simulink model "mc_pos"  (R2021a)
settings: Solver=FixedStepAuto  StartTime=0.0  StopTime=10.0  FixedStep=0.1  RelTol=1e-3
undefined symbols (not defined in the file): CONSTANTS_ONE_G, DiscIntNeverNeededParam, MPC_LAND_SPEED, MPC_SPOOLUP_TIME, MPC_THR_HOVER, MPC_THR_MAX, MPC_THR_MIN, MPC_TILTMAX_AIR, MPC_TILTMAX_LND, MPC_TKO_RAMP_T, MPC_VELD_LP, MPC_XY_P, MPC_XY_VEL_D_ACC, MPC_XY_VEL_I_ACC, MPC_XY_VEL_MAX, MPC_XY_VEL_P_ACC, MPC_Z_P, MPC_Z_VEL_D_ACC, MPC_Z_VEL_I_ACC, MPC_Z_VEL_MAX_DN, MPC_Z_VEL_MAX_UP, MPC_Z_VEL_P_ACC, PX4_TAKEOFF_STATUS, WV_EN
libraries: simulink x16, vrlib x2, sharedtransform x2, aerolibconvert2 x1
(part 1 of 3)
settings Model: DataDictionary=px4_dict.sldd  Creator=DELL  LastModifiedBy=yu
settings OptimizationCC: DefaultParameterBehavior=Inlined  EnhancedBackFolding=on  PassReuseOutputArgsAs=Individual arguments  ZeroExternalMemoryAtStartup=off  ZeroInternalMemoryAtStartup=off  OptimizeBlockOrder=speed  DifferentSizesBufferReuse=on  OptimizationCustomize=off  EfficientTunableParamExpr=on
settings DebuggingCC: ParameterTunabilityLossMsg=error
settings SFSimCC: MATLABDynamicMemAlloc=off
settings RTWCC: SystemTargetFile=ert.tlc  TemplateMakefile=ert_default_tmf
settings CodeAppCC: ForceParamTrailComments=on  IgnoreCustomStorageClasses=off  OperatorAnnotations=on  SimulinkDataObjDesc=on  SFDataObjDesc=on  InsertBlockDesc=on
settings ERTTargetCC: TargetLangStandard=C99 (ISO)  GenerateSampleERTMain=on  SupportContinuousTime=on  InlinedParameterPlacement=NonHierarchical  ERTCustomFileTemplate=example_file_process.tlc

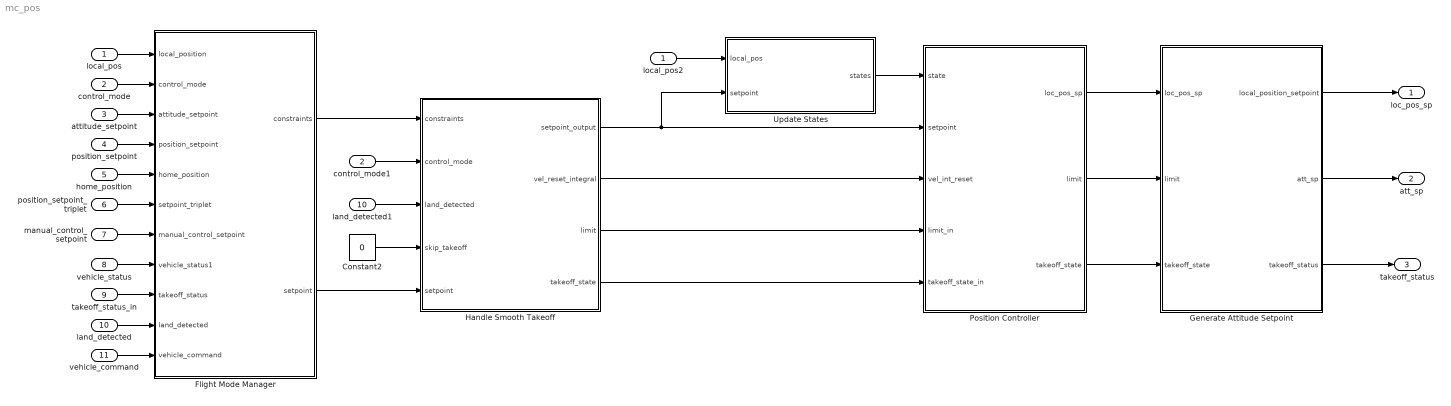
== system mc_pos ==
  local_pos : Inport  OutDataTypeStr=Bus: px4_vehicle_local_position
  control_mode : Inport  Port=2  OutDataTypeStr=Bus: px4_vehicle_control_mode
  attitude_setpoint : Inport  Port=3  OutDataTypeStr=Bus: px4_vehicle_attitude_setpoint
  position_setpoint : Inport  Port=4  OutDataTypeStr=Bus: px4_vehicle_local_position_setpoint
  home_position : Inport  Port=5  OutDataTypeStr=Bus: px4_home_position
  position_setpoint_triplet : Inport  Port=6  OutDataTypeStr=Bus: px4_position_setpoint_triplet
  manual_control_setpoint : Inport  Port=7  OutDataTypeStr=Bus: px4_manual_control_setpoint
  vehicle_status : Inport  Port=8  OutDataTypeStr=Bus: px4_vehicle_status
  takeoff_status_in : Inport  Port=9  OutDataTypeStr=Bus: px4_takeoff_status
  land_detected : Inport  Port=10  OutDataTypeStr=Bus: px4_vehicle_land_detected
  vehicle_command : Inport  Port=11  OutDataTypeStr=Bus: px4_vehicle_command
  Constant2 : Constant  Value=0  OutDataTypeStr=boolean
  Flight Mode Manager : Subsystem
  Generate Attitude Setpoint : Subsystem
  Handle Smooth Takeoff : Stateflow chart  TreatAsAtomicUnit=on
  Position Controller : Subsystem
  Update States : Subsystem
  control_mode1 : InportShadow  Port=2  OutDataTypeStr=Bus: px4_vehicle_control_mode
  land_detected1 : InportShadow  Port=10  OutDataTypeStr=Bus: px4_vehicle_land_detected
  local_pos2 : InportShadow  OutDataTypeStr=Bus: px4_vehicle_local_position
  loc_pos_sp : Outport  OutDataTypeStr=Bus: px4_vehicle_local_position_setpoint  BusOutputAsStruct=on
  att_sp : Outport  Port=2  OutDataTypeStr=Bus: px4_vehicle_attitude_setpoint  BusOutputAsStruct=on
  takeoff_status : Outport  Port=3  OutDataTypeStr=Bus: px4_takeoff_status  BusOutputAsStruct=on
  wires:
  local_pos/1 -> Flight Mode Manager/1(local_position)
  Flight Mode Manager/2(setpoint) -> Handle Smooth Takeoff/5(setpoint)
  Update States/1(states) -> Position Controller/1(state)
  Position Controller/1(loc_pos_sp) -> Generate Attitude Setpoint/1(loc_pos_sp)
  land_detected1/1 -> Handle Smooth Takeoff/3(land_detected)
  Flight Mode Manager/1(constraints) -> Handle Smooth Takeoff/1(constraints)
  Constant2/1 -> Handle Smooth Takeoff/4(skip_takeoff)
  Handle Smooth Takeoff/1(setpoint_output) -> Update States/2(setpoint), Position Controller/2(setpoint)
  Handle Smooth Takeoff/3(limit) -> Position Controller/4(limit_in)
  Handle Smooth Takeoff/2(vel_reset_integral) -> Position Controller/3(vel_int_reset)
  control_mode/1 -> Flight Mode Manager/2(control_mode)
  land_detected/1 -> Flight Mode Manager/10(land_detected)
  position_setpoint/1 -> Flight Mode Manager/4(position_setpoint)
  home_position/1 -> Flight Mode Manager/5(home_position)
  position_setpoint_triplet/1 -> Flight Mode Manager/6(setpoint_triplet)
  manual_control_setpoint/1 -> Flight Mode Manager/7(manual_control_setpoint)
  vehicle_status/1 -> Flight Mode Manager/8(vehicle_status1)
  Generate Attitude Setpoint/2(att_sp) -> att_sp/1
  attitude_setpoint/1 -> Flight Mode Manager/3(attitude_setpoint)
  takeoff_status_in/1 -> Flight Mode Manager/9(takeoff_status)
  local_pos2/1 -> Update States/1(local_pos)
  vehicle_command/1 -> Flight Mode Manager/11(vehicle_command)
  control_mode1/1 -> Handle Smooth Takeoff/2(control_mode)
  Position Controller/2(limit) -> Generate Attitude Setpoint/2(limit)
  Handle Smooth Takeoff/4(takeoff_state) -> Position Controller/5(takeoff_state_in)
  Position Controller/3(takeoff_state) -> Generate Attitude Setpoint/3(takeoff_state)
  Generate Attitude Setpoint/3(takeoff_status) -> takeoff_status/1
  Generate Attitude Setpoint/1(local_position_setpoint) -> loc_pos_sp/1

== system mc_pos/Flight Mode Manager ==
  local_position : Inport  OutDataTypeStr=Bus: px4_vehicle_local_position
  control_mode : Inport  Port=2  OutDataTypeStr=Bus: px4_vehicle_control_mode
  attitude_setpoint : Inport  Port=3  OutDataTypeStr=Bus: px4_vehicle_attitude_setpoint
  position_setpoint : Inport  Port=4  OutDataTypeStr=Bus: px4_vehicle_local_position_setpoint
  home_position : Inport  Port=5  OutDataTypeStr=Bus: px4_home_position
  setpoint_triplet : Inport  Port=6  OutDataTypeStr=Bus: px4_position_setpoint_triplet
  manual_control_setpoint : Inport  Port=7  OutDataTypeStr=Bus: px4_manual_control_setpoint
  vehicle_status1 : Inport  Port=8  OutDataTypeStr=Bus: px4_vehicle_status
  Bus Element In : Inport  Port=9  PortName=takeoff_status  Element=takeoff_state
  Bus Element In1 : Inport  Port=9  PortName=takeoff_status  Element=takeoff_state
  land_detected : Inport  Port=10  OutDataTypeStr=Bus: px4_vehicle_land_detected
  vehicle_command : Inport  Port=11  OutDataTypeStr=Bus: px4_vehicle_command
  Flight Task : Stateflow chart  TreatAsAtomicUnit=on
  Output : Subsystem
  Weather Vane : Subsystem
  control_mode1 : InportShadow  Port=2  OutDataTypeStr=Bus: px4_vehicle_control_mode
  home_position1 : InportShadow  Port=5  OutDataTypeStr=Bus: px4_home_position
  local_position1 : InportShadow  OutDataTypeStr=Bus: px4_vehicle_local_position
  local_position2 : InportShadow  OutDataTypeStr=Bus: px4_vehicle_local_position
  vehicle_status : InportShadow  Port=8  OutDataTypeStr=Bus: px4_vehicle_status
  constraints : Outport
  setpoint : Outport  Port=2
  wires:
  home_position/1 -> Flight Task/5(home_position)
  setpoint_triplet/1 -> Flight Task/6(triplet_setpoint)
  manual_control_setpoint/1 -> Flight Task/7(manual_control_setpoint)
  vehicle_status1/1 -> Flight Task/8(vehicle_status)
  attitude_setpoint/1 -> Weather Vane/3(attitude_setpoint)
  Weather Vane/1(weather_vane) -> Flight Task/1(weather_vane)
  position_setpoint/1 -> Flight Task/2(position_setpoint_input)
  Flight Task/4(acceleration_setpoint) -> Output/3(acceleration_setpoint)
  Flight Task/5(jerk_setpoint) -> Output/4(jerk_setpoint)
  Flight Task/3(velocity_setpoint) -> Output/2(velocity_setpoint)
  Flight Task/6(yaw_setpoint) -> Output/5(yaw_setpoint)
  Flight Task/2(position_setpoint) -> Output/1(position_setpoint)
  Flight Task/7(yawspeed_setpoint) -> Output/6(yawspeed_setpoint)
  Flight Task/1(constraints) -> constraints/1
  control_mode1/1 -> Flight Task/3(control_mode)
  control_mode/1 -> Weather Vane/2(control_mode)
  local_position1/1 -> Flight Task/4(local_position)
  local_position/1 -> Weather Vane/1(local_position)
  land_detected/1 -> Output/9(land_detect)
  home_position1/1 -> Output/8(home_position)
  local_position2/1 -> Output/7(local_position)
  Bus Element In/1 -> Flight Task/9(takeoff_state)
  Bus Element In1/1 -> Output/10(takeoff_status)
  vehicle_status/1 -> Weather Vane/4(vehicle_status)
  Output/1(setpoint) -> setpoint/1
  vehicle_command/1 -> Flight Task/10(vehicle_command)

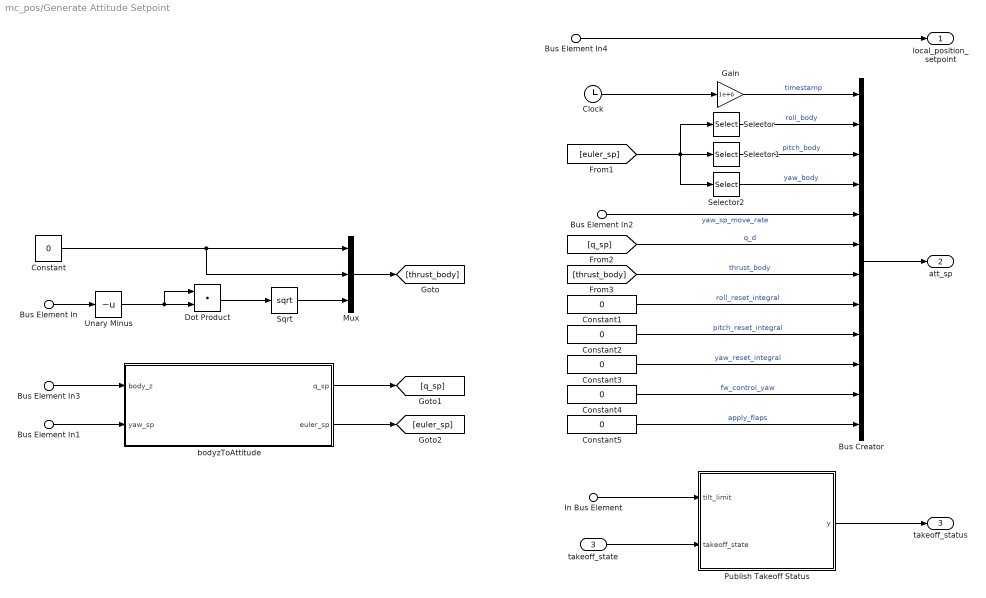
== system mc_pos/Generate Attitude Setpoint ==
  Bus Element In4 : Inport  PortName=loc_pos_sp
  Bus Element In1 : Inport  PortName=loc_pos_sp  Element=yaw
  Bus Element In2 : Inport  PortName=loc_pos_sp  Element=yawspeed
  Bus Element In : Inport  PortName=loc_pos_sp  Element=thrust
  Bus Element In3 : Inport  PortName=loc_pos_sp  Element=thrust
  In Bus Element : Inport  Port=2  PortName=limit
  takeoff_state : Inport  Port=3
  Bus Creator : BusCreator  Inputs=12
  Clock : Clock
  Constant : Constant  Value=0  OutDataTypeStr=single
  Constant{1..4} (4 alike) : Constant  Value=0  OutDataTypeStr=boolean
  Constant5 : Constant  Value=0  OutDataTypeStr=uint8
  Dot Product : DotProduct  InputSameDT=on  OutDataTypeStr=Inherit: Inherit via internal rule
  Gain : Gain  Gain=1e+6  OutDataTypeStr=uint64
      settings: AttributesFormatString=%<Gain>
  Mux : Mux  Inputs=3
  Publish Takeoff Status : Subsystem
  Selector : Selector  InputPortWidth=3  IndexOptions=Index vector (dialog)  Indices=3  OutputSizes=1
  Selector1 : Selector  InputPortWidth=3  IndexOptions=Index vector (dialog)  Indices=2  OutputSizes=1
  Selector2 : Selector  InputPortWidth=3  IndexOptions=Index vector (dialog)  Indices=1  OutputSizes=1
  Sqrt : Sqrt  SaturateOnIntegerOverflow=on
  Unary Minus : UnaryMinus
  bodyzToAttitude : Subsystem
  local_position_setpoint : Outport  OutDataTypeStr=Bus: px4_vehicle_local_position_setpoint
  att_sp : Outport  Port=2  OutDataTypeStr=Bus: px4_vehicle_attitude_setpoint
  takeoff_status : Outport  Port=3  OutDataTypeStr=Bus: px4_takeoff_status
  wires:
  Bus Creator/1 -> att_sp/1
  Bus Element In2/1 -> Bus Creator/5  "yaw_sp_move_rate"
  Bus Element In/1 -> Unary Minus/1
  Unary Minus/1 -> Dot Product/1, Dot Product/2
  Dot Product/1 -> Sqrt/1
  Sqrt/1 -> Mux/3
  Bus Element In3/1 -> bodyzToAttitude/1(body_z)
  Bus Element In1/1 -> bodyzToAttitude/2(yaw_sp)
  bodyzToAttitude/1(q_sp) -> [q_sp]
  Constant/1 -> Mux/2, Mux/1
  Mux/1 -> [thrust_body]
  Selector/1 -> Bus Creator/2  "roll_body"
  Selector1/1 -> Bus Creator/3  "pitch_body"
  Selector2/1 -> Bus Creator/4  "yaw_body"
  [q_sp] -> Bus Creator/6  "q_d"
  [thrust_body] -> Bus Creator/7  "thrust_body"
  bodyzToAttitude/2(euler_sp) -> [euler_sp]
  [euler_sp] -> Selector2/1, Selector/1, Selector1/1
  Clock/1 -> Gain/1
  Constant1/1 -> Bus Creator/8  "roll_reset_integral"
  Constant2/1 -> Bus Creator/9  "pitch_reset_integral"
  Constant3/1 -> Bus Creator/10  "yaw_reset_integral"
  Constant4/1 -> Bus Creator/11  "fw_control_yaw"
  Constant5/1 -> Bus Creator/12  "apply_flaps"
  Gain/1 -> Bus Creator/1  "timestamp"
  Bus Element In4/1 -> local_position_setpoint/1
  In Bus Element/1 -> Publish Takeoff Status/1(tilt_limit)
  takeoff_state/1 -> Publish Takeoff Status/2(takeoff_state)
  Publish Takeoff Status/1(y) -> takeoff_status/1

== system mc_pos/Handle Smooth Takeoff/UpdateTakeoffState.tilt_limit_slew_rate_update ==
  input : Inport  OutDataTypeStr=double  PortDimensions=1
  f : TriggerPort  TriggerType=function-call  VariantControl=(inherit)
      settings: CopyFcn=Stateflow.SLINSF.SimulinkMan.removeBlockPreDeleteFcn  PreDeleteFcn=Stateflow.SLINSF.SimulinkMan.unsafePredeleteFcn
  Angle Conversion : aerolibconvert2/Angle Conversion  IU=deg  OU=rad
  Data Type Conversion : DataTypeConversion  OutDataTypeStr=single
  Delay One Step : Delay  DelayLength=1
  Gain : Gain  OutDataTypeStr=single
  Saturation Dynamic : simulink/Discontinuities/Saturation Dynamic  OutMin=[]  OutMax=[]  OutDataTypeStr=single  OutputDataTypeScalingMode=single  OutDataType=fixdt(1, 16)  OutScaling=2^-10  DoSatur=off
  Sum : Sum  Inputs=|+-
  Sum1 : Sum  Inputs=|++
  Unary Minus1 : UnaryMinus
  Weighted Sample Time : SampleTimeMath  TsampMathOp=*  OutDataTypeStr=Inherit: Inherit via back propagation
  slew_rate : Constant  Value=0.2  OutDataTypeStr=single
  result : Outport
  wires:
  Sum/1 -> Saturation Dynamic/2  "dvalue_desired"
  Unary Minus1/1 -> Saturation Dynamic/3
  Saturation Dynamic/1 -> Sum1/1  "dvalue"
  Delay One Step/1 -> Sum/2, Sum1/2
  slew_rate/1 -> Weighted Sample Time/1
  input/1 -> Angle Conversion/1
  Angle Conversion/1 -> Data Type Conversion/1
  Weighted Sample Time/1 -> Unary Minus1/1, Saturation Dynamic/1  "dvalue_max"
  Sum1/1 -> Gain/1, Delay One Step/1
  Data Type Conversion/1 -> Sum/1
  Gain/1 -> result/1

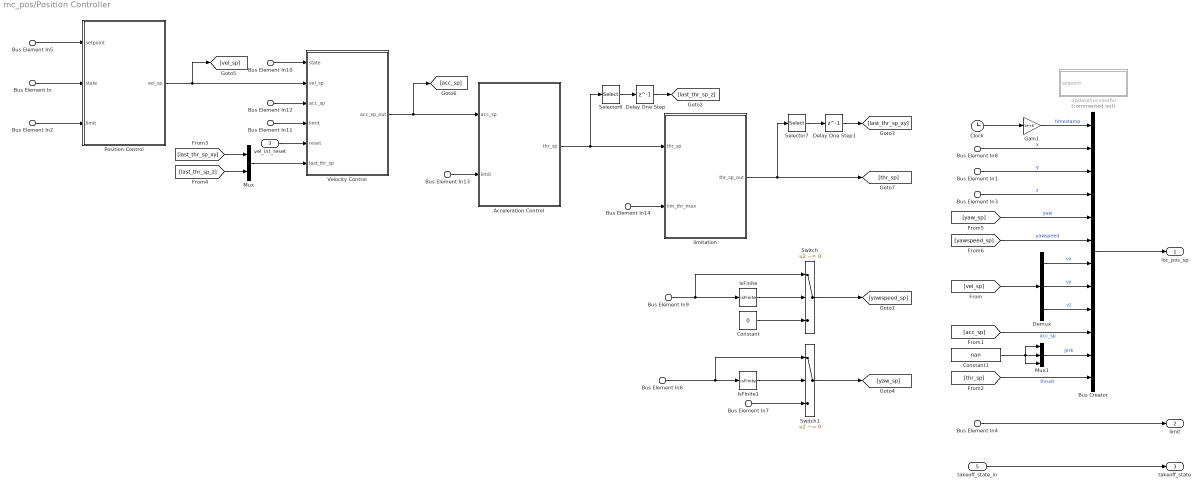
== system mc_pos/Position Controller ==
  Bus Element In : Inport  PortName=state
  Bus Element In10 : Inport  PortName=state
  Bus Element In7 : Inport  PortName=state  Element=yaw
  Bus Element In5 : Inport  Port=2  PortName=setpoint
  Bus Element In12 : Inport  Port=2  PortName=setpoint  Element=acceleration
  Bus Element In9 : Inport  Port=2  PortName=setpoint  Element=yawspeed
  Bus Element In6 : Inport  Port=2  PortName=setpoint  Element=yaw
  Bus Element In8 : Inport  Port=2  PortName=setpoint  Element=x
  Bus Element In1 : Inport  Port=2  PortName=setpoint  Element=y
  Bus Element In3 : Inport  Port=2  PortName=setpoint  Element=z
  vel_int_reset : Inport  Port=3
  Bus Element In{2,4,11,13} (4 alike) : Inport  Port=4  PortName=limit_in
  Bus Element In14 : Inport  Port=4  PortName=limit_in  Element=lim_thr_max
  takeoff_state_in : Inport  Port=5
  Acceleration Control : Subsystem
  Bus Creator : BusCreator  Inputs=12
  Clock : Clock
  Constant : Constant  Value=0  OutDataTypeStr=single
  Constant1 : Constant  Value=nan  OutDataTypeStr=single
  Delay One Step : Delay  DelayLength=1
  Delay One Step1 : Delay  DelayLength=1
  Demux : Demux  Outputs=3
  Gain1 : Gain  Gain=1e+6  OutDataTypeStr=uint64
      settings: AttributesFormatString=%<Gain>
  IsFinite : RelationalOperator  Operator=isFinite  OutDataTypeStr=boolean  RndMeth=Simplest
  IsFinite1 : RelationalOperator  Operator=isFinite  OutDataTypeStr=boolean  RndMeth=Simplest
  Mux : Mux  Inputs=2
  Mux1 : Mux  Inputs=3
  Position Control : Subsystem
  Selector6 : Selector  InputPortWidth=3  IndexOptions=Index vector (dialog)  Indices=3  OutputSizes=1
  Selector7 : Selector  InputPortWidth=3  IndexOptions=Index vector (dialog)  Indices=[1 2]  OutputSizes=1
  Switch : Switch  Criteria=u2 ~= 0
  Switch1 : Switch  Criteria=u2 ~= 0
  Velocity Control : Subsystem
  limitation : Subsystem
  updateSuccessful : Subsystem  Commented=on
  loc_pos_sp : Outport
  limit : Outport  Port=2
  takeoff_state : Outport  Port=3
  wires:
  Bus Element In5/1 -> Position Control/1(setpoint)
  Bus Element In/1 -> Position Control/2(state)
  Bus Element In2/1 -> Position Control/3(limit)
  Position Control/1(vel_sp) -> [vel_sp], Velocity Control/2(vel_sp)
  Bus Element In10/1 -> Velocity Control/1(state)
  Bus Element In11/1 -> Velocity Control/4(limit)
  [last_thr_sp_xy] -> Mux/1
  Mux/1 -> Velocity Control/6(last_thr_sp)
  [last_thr_sp_z] -> Mux/2
  Bus Element In12/1 -> Velocity Control/3(acc_sp)
  Velocity Control/1(acc_sp_out) -> [acc_sp], Acceleration Control/1(acc_sp)
  Bus Element In13/1 -> Acceleration Control/2(limit)
  Selector6/1 -> Delay One Step/1
  Acceleration Control/1(thr_sp) -> limitation/1(thr_sp), Selector6/1
  Bus Element In14/1 -> limitation/2(lim_thr_max)
  Selector7/1 -> Delay One Step1/1
  limitation/1(thr_sp_out) -> Selector7/1, [thr_sp]
  Bus Element In9/1 -> Switch/1, IsFinite/1
  IsFinite/1 -> Switch/2
  Constant/1 -> Switch/3
  Switch/1 -> [yawspeed_sp]
  Bus Element In6/1 -> IsFinite1/1, Switch1/1
  IsFinite1/1 -> Switch1/2
  Bus Element In7/1 -> Switch1/3
  Switch1/1 -> [yaw_sp]
  [thr_sp] -> Bus Creator/12  "thrust"
  [yaw_sp] -> Bus Creator/5  "yaw"
  [yawspeed_sp] -> Bus Creator/6  "yawspeed"
  [acc_sp] -> Bus Creator/10  "acc_sp"
  Bus Element In8/1 -> Bus Creator/2  "x"
  Bus Element In1/1 -> Bus Creator/3  "y"
  Bus Element In3/1 -> Bus Creator/4  "z"
  vel_int_reset/1 -> Velocity Control/5(reset)
  [vel_sp] -> Demux/1
  Demux/1 -> Bus Creator/7  "vx"
  Demux/2 -> Bus Creator/8  "vy"
  Demux/3 -> Bus Creator/9  "vz"
  Constant1/1 -> Mux1/2, Mux1/3, Mux1/1
  Mux1/1 -> Bus Creator/11  "jerk"
  Bus Creator/1 -> loc_pos_sp/1
  Gain1/1 -> Bus Creator/1  "timestamp"
  Clock/1 -> Gain1/1
  Bus Element In4/1 -> limit/1
  takeoff_state_in/1 -> takeoff_state/1
  Delay One Step/1 -> [last_thr_sp_z]
  Delay One Step1/1 -> [last_thr_sp_xy]

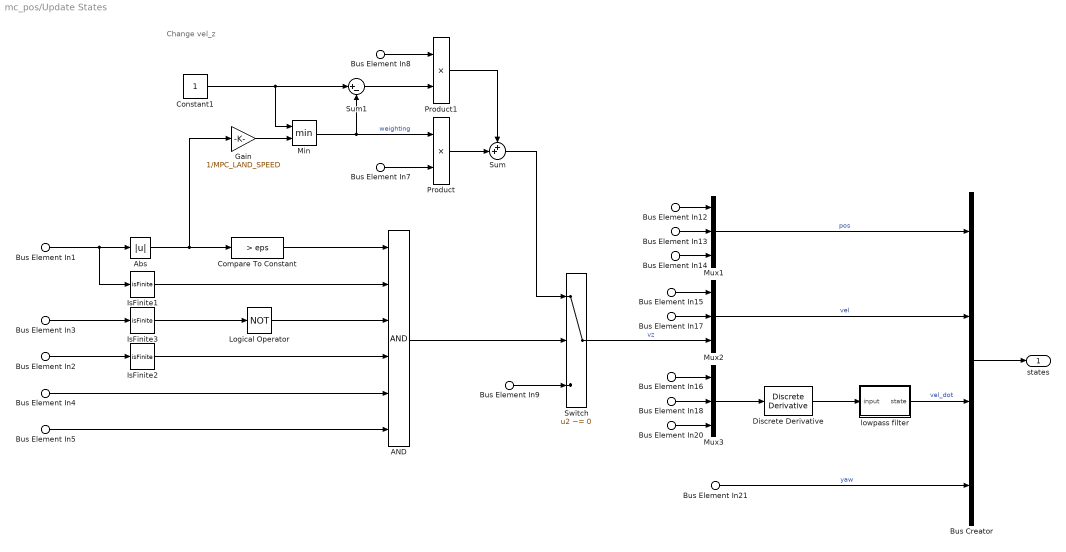
== system mc_pos/Update States ==
  note: Change vel_z
  Bus Element In2 : Inport  PortName=local_pos  Element=z_deriv
  Bus Element In7 : Inport  PortName=local_pos  Element=z_deriv
  Bus Element In4 : Inport  PortName=local_pos  Element=z_valid
  Bus Element In5 : Inport  PortName=local_pos  Element=v_z_valid
  Bus Element In8 : Inport  PortName=local_pos  Element=vz
  Bus Element In20 : Inport  PortName=local_pos  Element=vz
  Bus Element In9 : Inport  PortName=local_pos  Element=vz
  Bus Element In12 : Inport  PortName=local_pos  Element=x
  Bus Element In13 : Inport  PortName=local_pos  Element=y
  Bus Element In14 : Inport  PortName=local_pos  Element=z
  Bus Element In15 : Inport  PortName=local_pos  Element=vx
  Bus Element In16 : Inport  PortName=local_pos  Element=vx
  Bus Element In17 : Inport  PortName=local_pos  Element=vy
  Bus Element In18 : Inport  PortName=local_pos  Element=vy
  Bus Element In21 : Inport  PortName=local_pos  Element=heading
  Bus Element In1 : Inport  Port=2  PortName=setpoint  Element=vz
  Bus Element In3 : Inport  Port=2  PortName=setpoint  Element=z
  AND : Logic  Inputs=6  AllPortsSameDT=off  OutDataTypeStr=boolean
  Abs : Abs
  Bus Creator : BusCreator  Inputs=4
  Compare To Constant : simulink/Logic and Bit Operations/Compare To Constant  relop=>  const=eps  OutDataTypeStr=boolean
      settings: AttributesFormatString=%<relop> %<const>
  Constant1 : Constant  OutDataTypeStr=single
  Discrete Derivative : simulink/Discrete/Discrete Derivative  gainval=1.0  ICPrevScaledInput=0.0  OutMin=[]  OutMax=[]  OutDataType=fixdt(1, 16)  OutScaling=2^-10  DoSatur=off
  Gain : Gain  Gain=1/MPC_LAND_SPEED
      settings: AttributesFormatString=%<Gain>
  IsFinite1 : RelationalOperator  Operator=isFinite  OutDataTypeStr=boolean  RndMeth=Simplest
  IsFinite2 : RelationalOperator  Operator=isFinite  OutDataTypeStr=boolean  RndMeth=Simplest
  IsFinite3 : RelationalOperator  Operator=isFinite  OutDataTypeStr=boolean  RndMeth=Simplest
  Logical Operator : Logic  Operator=NOT  AllPortsSameDT=off  OutDataTypeStr=boolean
  Min : MinMax  Inputs=2
  Mux1 : Mux  Inputs=3
  Mux2 : Mux  Inputs=3
  Mux3 : Mux  Inputs=3
  Product : Product
  Product1 : Product
  Sum : Sum  Inputs=++|
  Sum1 : Sum  Inputs=|+-
  Switch : Switch  Criteria=u2 ~= 0
  lowpass filter : Subsystem
  states : Outport
  wires:
  Bus Element In1/1 -> IsFinite1/1, Abs/1
  Abs/1 -> Gain/1, Compare To Constant/1
  Bus Element In2/1 -> IsFinite2/1
  AND/1 -> Switch/2
  Bus Element In9/1 -> Switch/3
  Gain/1 -> Min/2
  Constant1/1 -> Sum1/1, Min/1
  Min/1 -> Sum1/2, Product/1  "weighting"
  Bus Element In7/1 -> Product/2
  Product/1 -> Sum/2
  Sum/1 -> Switch/1
  Sum1/1 -> Product1/2
  Bus Element In8/1 -> Product1/1
  Product1/1 -> Sum/1
  Mux1/1 -> Bus Creator/1  "pos"
  Mux2/1 -> Bus Creator/2  "vel"
  lowpass filter/1(state) -> Bus Creator/3  "vel_dot"
  Bus Element In21/1 -> Bus Creator/4  "yaw"
  Bus Creator/1 -> states/1
  Bus Element In15/1 -> Mux2/1
  Bus Element In20/1 -> Mux3/3
  Discrete Derivative/1 -> lowpass filter/1(input)
  Switch/1 -> Mux2/3  "vz"
  Mux3/1 -> Discrete Derivative/1
  Bus Element In12/1 -> Mux1/1
  Bus Element In18/1 -> Mux3/2
  Bus Element In16/1 -> Mux3/1
  Bus Element In13/1 -> Mux1/2
  Bus Element In17/1 -> Mux2/2
  Bus Element In14/1 -> Mux1/3
  Compare To Constant/1 -> AND/1
  IsFinite2/1 -> AND/4
  IsFinite1/1 -> AND/2
  Bus Element In4/1 -> AND/5
  Bus Element In5/1 -> AND/6
  IsFinite3/1 -> Logical Operator/1
  Bus Element In3/1 -> IsFinite3/1
  Logical Operator/1 -> AND/3

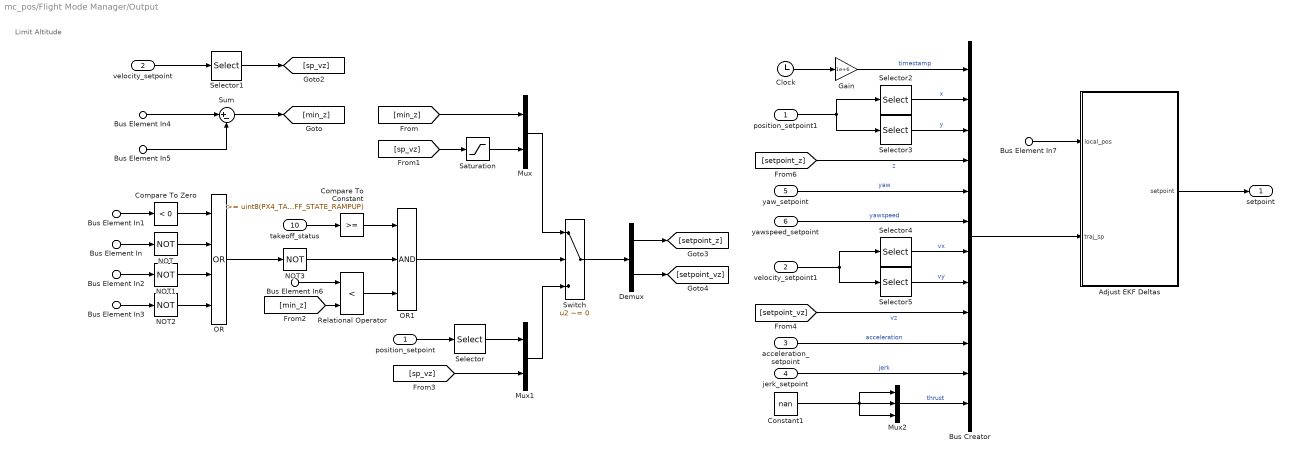
== system mc_pos/Flight Mode Manager/Output ==
  note: Limit Altitude
  position_setpoint : Inport
  velocity_setpoint : Inport  Port=2
  acceleration_setpoint : Inport  Port=3
  jerk_setpoint : Inport  Port=4
  yaw_setpoint : Inport  Port=5
  yawspeed_setpoint : Inport  Port=6
  Bus Element In7 : Inport  Port=7  PortName=local_position
  Bus Element In2 : Inport  Port=7  PortName=local_position  Element=z_valid
  Bus Element In3 : Inport  Port=7  PortName=local_position  Element=v_z_valid
  Bus Element In6 : Inport  Port=7  PortName=local_position  Element=z
  Bus Element In : Inport  Port=8  PortName=home_position  Element=valid_alt
  Bus Element In4 : Inport  Port=8  PortName=home_position  Element=z
  Bus Element In1 : Inport  Port=9  PortName=land_detect  Element=alt_max
  Bus Element In5 : Inport  Port=9  PortName=land_detect  Element=alt_max
  takeoff_status : Inport  Port=10
  Adjust EKF Deltas : Subsystem
  Bus Creator : BusCreator  Inputs=12
  Clock : Clock
  Compare To Constant : simulink/Logic and Bit Operations/Compare To Constant  relop=>=  const=uint8(PX4_TAKEOFF_STATUS.TAKEOFF_STATE_RAMPUP)  OutDataTypeStr=boolean
  Compare To Zero : simulink/Logic and Bit Operations/Compare To Zero  relop=<  OutDataTypeStr=boolean
  Constant1 : Constant  Value=nan  OutDataTypeStr=single
  Demux : Demux  Outputs=2
  Gain : Gain  Gain=1e+6  OutDataTypeStr=uint64
      settings: AttributesFormatString=%<Gain>
  Mux : Mux  Inputs=2
  Mux1 : Mux  Inputs=2
  Mux2 : Mux  Inputs=3
  NOT{,1..3} (4 alike) : Logic  Operator=NOT  AllPortsSameDT=off  OutDataTypeStr=boolean
  OR : Logic  Operator=OR  Inputs=4  AllPortsSameDT=off  OutDataTypeStr=boolean
  OR1 : Logic  Inputs=3  AllPortsSameDT=off  OutDataTypeStr=boolean
  Relational Operator : RelationalOperator  Operator=<  OutDataTypeStr=boolean  RndMeth=Simplest
  Saturation : Saturate  UpperLimit=inf  LowerLimit=0.0
      settings: AttributesFormatString=[%<LowerLimit>, %<UpperLimit>]
  Selector : Selector  InputPortWidth=3  IndexOptions=Index vector (dialog)  Indices=3  OutputSizes=1
  Selector1 : Selector  InputPortWidth=3  IndexOptions=Index vector (dialog)  Indices=3  OutputSizes=1
  Selector2 : Selector  InputPortWidth=3  IndexOptions=Index vector (dialog)  Indices=1  OutputSizes=1
  Selector3 : Selector  InputPortWidth=3  IndexOptions=Index vector (dialog)  Indices=2  OutputSizes=1
  Selector4 : Selector  InputPortWidth=3  IndexOptions=Index vector (dialog)  Indices=1  OutputSizes=1
  Selector5 : Selector  InputPortWidth=3  IndexOptions=Index vector (dialog)  Indices=2  OutputSizes=1
  Sum : Sum  Inputs=|+-
  Switch : Switch  Criteria=u2 ~= 0
  position_setpoint1 : InportShadow
  velocity_setpoint1 : InportShadow  Port=2
  setpoint : Outport
  wires:
  position_setpoint/1 -> Selector/1
  velocity_setpoint/1 -> Selector1/1
  Selector1/1 -> [sp_vz]
  Bus Element In1/1 -> Compare To Zero/1
  Compare To Zero/1 -> OR/1
  Bus Element In/1 -> NOT/1
  NOT/1 -> OR/2
  Bus Element In2/1 -> NOT1/1
  NOT1/1 -> OR/3
  Bus Element In3/1 -> NOT2/1
  NOT2/1 -> OR/4
  OR/1 -> NOT3/1
  NOT3/1 -> OR1/2
  Bus Element In4/1 -> Sum/1
  Bus Element In5/1 -> Sum/2
  Bus Element In6/1 -> Relational Operator/1
  Sum/1 -> [min_z]
  Relational Operator/1 -> OR1/3
  OR1/1 -> Switch/2
  Mux/1 -> Switch/1
  [min_z] -> Mux/1
  Mux1/1 -> Switch/3
  Selector/1 -> Mux1/1
  [sp_vz] -> Mux1/2
  Switch/1 -> Demux/1
  Demux/1 -> [setpoint_z]
  Demux/2 -> [setpoint_vz]
  position_setpoint1/1 -> Selector2/1, Selector3/1
  Selector2/1 -> Bus Creator/2  "x"
  Selector3/1 -> Bus Creator/3  "y"
  [setpoint_z] -> Bus Creator/4  "z"
  velocity_setpoint1/1 -> Selector4/1, Selector5/1
  Selector4/1 -> Bus Creator/7  "vx"
  Selector5/1 -> Bus Creator/8  "vy"
  [setpoint_vz] -> Bus Creator/9  "vz"
  yaw_setpoint/1 -> Bus Creator/5  "yaw"
  yawspeed_setpoint/1 -> Bus Creator/6  "yawspeed"
  acceleration_setpoint/1 -> Bus Creator/10  "acceleration"
  jerk_setpoint/1 -> Bus Creator/11  "jerk"
  Constant1/1 -> Mux2/3, Mux2/1, Mux2/2
  Mux2/1 -> Bus Creator/12  "thrust"
  Clock/1 -> Gain/1
  Bus Creator/1 -> Adjust EKF Deltas/2(traj_sp)
  Gain/1 -> Bus Creator/1  "timestamp"
  Compare To Constant/1 -> OR1/1
  takeoff_status/1 -> Compare To Constant/1
  [min_z] -> Relational Operator/2
  Bus Element In7/1 -> Adjust EKF Deltas/1(local_pos)
  Adjust EKF Deltas/1(setpoint) -> setpoint/1
  Saturation/1 -> Mux/2
  [sp_vz] -> Saturation/1

== system mc_pos/Flight Mode Manager/Weather Vane ==
  Bus Element In3 : Inport  PortName=local_position  Element=heading
  Bus Element In : Inport  Port=2  PortName=control_mode  Element=flag_control_manual_enabled
  Bus Element In4 : Inport  Port=2  PortName=control_mode  Element=flag_control_position_enabled
  Bus Element In2 : Inport  Port=3  PortName=attitude_setpoint  Element=q_d
  In Bus Element : Inport  Port=4  PortName=vehicle_status  Element=is_vtol
  Bus Creator : BusCreator  Inputs=3
  Constant2 : Constant  Value=WV_EN  OutDataTypeStr=boolean
  Data Type Conversion1 : DataTypeConversion  OutDataTypeStr=boolean
  Product1 : Product  Inputs=4
  dcm_z : Subsystem
  weather_vane : Outport
  wires:
  Product1/1 -> Data Type Conversion1/1
  Bus Element In2/1 -> dcm_z/1(Q)
  dcm_z/1(out) -> Bus Creator/3  "dcm_z_sp_prev"
  Bus Element In3/1 -> Bus Creator/2  "yaw"
  Bus Creator/1 -> weather_vane/1
  Bus Element In/1 -> Product1/2
  In Bus Element/1 -> Product1/1
  Bus Element In4/1 -> Product1/3
  Constant2/1 -> Product1/4
  Data Type Conversion1/1 -> Bus Creator/1  "is_active"

== system mc_pos/Generate Attitude Setpoint/Publish Takeoff Status ==
  tilt_limit : Inport  PortDimensions=1
  takeoff_state : Inport  Port=2  PortDimensions=1
  Bus Creator : BusCreator  Inputs=3
  Bus Selector : BusSelector  OutputSignals=takeoff_state
  Bus Selector1 : BusSelector  OutputSignals=lim_tilt
  Bus Selector2 : BusSelector  OutputSignals=lim_tilt
  Bus Selector3 : BusSelector  OutputSignals=lim_tilt
  Clock : Clock
  Constant : Constant  Value=1e-4  OutDataTypeStr=single
  Delay One Step : Delay  DelayLength=1
  Gain : Gain  Gain=1e+6  OutDataTypeStr=uint64
      settings: AttributesFormatString=%<Gain>
  MATLAB Function : MATLAB Function  TreatAsAtomicUnit=on
  NOT : Logic  Operator=NOT  AllPortsSameDT=off  OutDataTypeStr=boolean
  NOT1 : Logic  Operator=OR  AllPortsSameDT=off  OutDataTypeStr=boolean
  Relational Operator : RelationalOperator  Operator=~=  OutDataTypeStr=boolean  RndMeth=Simplest
  Switch : Switch  Criteria=u2 ~= 0
  takeoff_state1 : InportShadow  Port=2  PortDimensions=1
  tilt_limit1 : InportShadow  PortDimensions=1
  y : Outport
  wires:
  Bus Selector/1 -> Relational Operator/2  "<takeoff_state>"
  [y_last] -> Bus Selector1/1
  tilt_limit/1 -> Bus Selector2/1
  MATLAB Function/1(result) -> NOT/1
  Bus Selector1/1 -> MATLAB Function/2(y)  "<lim_tilt>"
  Delay One Step/1 -> [y_last]
  Bus Creator/1 -> Switch/1
  Switch/1 -> Delay One Step/1, y/1
  takeoff_state/1 -> Relational Operator/1  "takeoff_state"
  [y_last] -> Bus Selector/1
  NOT1/1 -> Switch/2
  takeoff_state1/1 -> Bus Creator/2  "takeoff_state"
  Gain/1 -> Bus Creator/1  "timestamp"
  Relational Operator/1 -> NOT1/1
  Clock/1 -> Gain/1
  NOT/1 -> NOT1/2
  Constant/1 -> MATLAB Function/3(eps_value)
  Bus Selector2/1 -> MATLAB Function/1(x)  "<lim_tilt>"
  tilt_limit1/1 -> Bus Selector3/1
  Bus Selector3/1 -> Bus Creator/3  "<lim_tilt>"
  [y_last] -> Switch/3

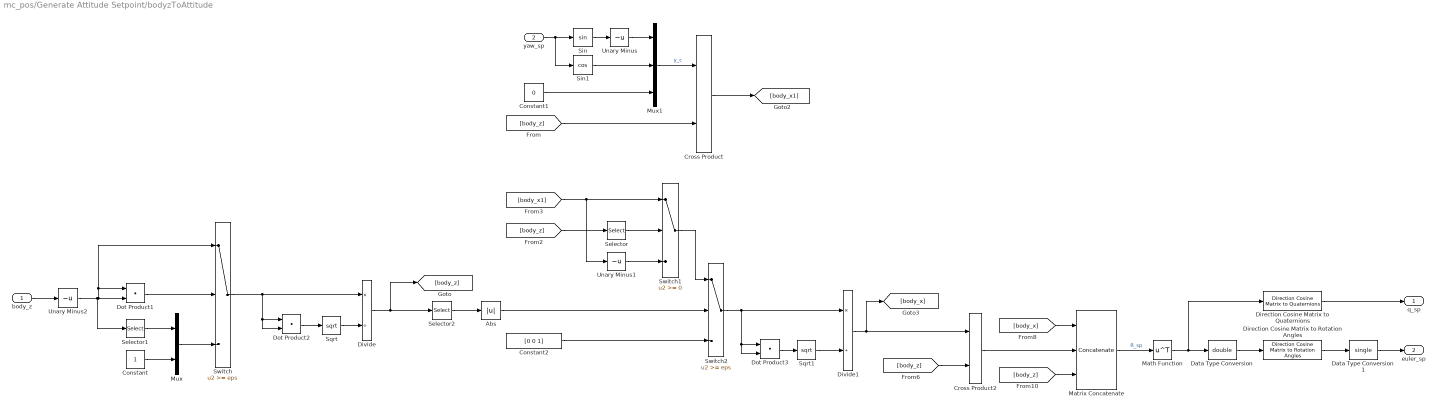
== system mc_pos/Generate Attitude Setpoint/bodyzToAttitude ==
  body_z : Inport
  yaw_sp : Inport  Port=2
  Abs : Abs
  Constant : Constant  OutDataTypeStr=single
  Constant1 : Constant  Value=0  OutDataTypeStr=single
  Constant2 : Constant  Value=[0 0 1]  OutDataTypeStr=single
  Cross Product : vrlib/Utilities/Cross Product
  Cross Product2 : vrlib/Utilities/Cross Product
  Data Type Conversion : DataTypeConversion  OutDataTypeStr=double
  Data Type Conversion1 : DataTypeConversion  OutDataTypeStr=single
  Direction Cosine Matrix to Rotation Angles : sharedtransform/Direction Cosine Matrix to Rotation Angles  rotationOrder=ZYX  aMode=aMode  action=None  tolerance=eps(2)
      settings: SourceProductBaseCode=AE,PW,DR,MT,UV,VE
  Direction Cosine Matrix to Quaternions : sharedtransform/Direction Cosine Matrix  to Quaternions  aMode=0  action=None  tolerance=eps(2)
      settings: SourceProductBaseCode=AE,PW,DR,MT,UV,VE
  Divide : Product  Inputs=*/
  Divide1 : Product  Inputs=*/
  Dot Product1 : DotProduct  InputSameDT=on  OutDataTypeStr=Inherit: Inherit via internal rule
  Dot Product2 : DotProduct  InputSameDT=on  OutDataTypeStr=Inherit: Inherit via internal rule
  Dot Product3 : DotProduct  InputSameDT=on  OutDataTypeStr=Inherit: Inherit via internal rule
  Math Function : Math  Operator=transpose  SaturateOnIntegerOverflow=on
  Matrix Concatenate : Concatenate  NumInputs=3  Mode=Multidimensional array  ConcatenateDimension=2
  Mux : Mux  Inputs=2
  Mux1 : Mux  Inputs=3
  Selector : Selector  InputPortWidth=3  IndexOptions=Index vector (dialog)  Indices=3  OutputSizes=1
  Selector1 : Selector  InputPortWidth=3  IndexOptions=Index vector (dialog)  Indices=[1 2]  OutputSizes=1
  Selector2 : Selector  InputPortWidth=3  IndexOptions=Index vector (dialog)  Indices=3  OutputSizes=1
  Sin : Trigonometry
  Sin1 : Trigonometry  Operator=cos
  Sqrt : Sqrt  SaturateOnIntegerOverflow=on
  Sqrt1 : Sqrt  SaturateOnIntegerOverflow=on
  Switch : Switch  Threshold=eps
      settings: AttributesFormatString=|
      | %<Criteria>
      | %<Threshold>
  Switch1 : Switch
      settings: AttributesFormatString=|
      | %<Criteria>
      | %<Threshold>
  Switch2 : Switch  Threshold=eps
      settings: AttributesFormatString=|
      | %<Criteria>
      | %<Threshold>
  Unary Minus : UnaryMinus
  Unary Minus1 : UnaryMinus
  Unary Minus2 : UnaryMinus
  q_sp : Outport
  euler_sp : Outport  Port=2
  wires:
  Dot Product1/1 -> Switch/2
  Mux/1 -> Switch/3
  Selector1/1 -> Mux/1
  body_z/1 -> Unary Minus2/1
  Constant/1 -> Mux/2
  Switch/1 -> Dot Product2/2, Dot Product2/1, Divide/1
  Dot Product2/1 -> Sqrt/1
  Sqrt/1 -> Divide/2
  yaw_sp/1 -> Sin1/1, Sin/1
  Sin/1 -> Unary Minus/1
  Unary Minus/1 -> Mux1/1
  Sin1/1 -> Mux1/2
  Constant1/1 -> Mux1/3
  Mux1/1 -> Cross Product/1  "y_c"
  [body_z] -> Cross Product/2
  Cross Product/1 -> [body_x1]
  Selector/1 -> Switch1/2
  [body_z] -> Selector/1
  Unary Minus1/1 -> Switch1/3
  [body_x1] -> Unary Minus1/1, Switch1/1
  Abs/1 -> Switch2/2
  Selector2/1 -> Abs/1
  Divide/1 -> Selector2/1, [body_z]
  Switch2/1 -> Divide1/1, Dot Product3/2, Dot Product3/1
  Sqrt1/1 -> Divide1/2
  Dot Product3/1 -> Sqrt1/1
  Divide1/1 -> [body_x], Cross Product2/1
  Matrix Concatenate/1 -> Math Function/1  "R_sp"
  Direction Cosine Matrix to Rotation Angles/1 -> Data Type Conversion1/1
  Math Function/1 -> Direction Cosine Matrix to Quaternions/1, Data Type Conversion/1
  Direction Cosine Matrix to Quaternions/1 -> q_sp/1
  [body_x] -> Matrix Concatenate/1
  Cross Product2/1 -> Matrix Concatenate/2
  [body_z] -> Matrix Concatenate/3
  Data Type Conversion/1 -> Direction Cosine Matrix to Rotation Angles/1
  Data Type Conversion1/1 -> euler_sp/1
  Unary Minus2/1 -> Dot Product1/2, Switch/1, Dot Product1/1, Selector1/1
  Constant2/1 -> Switch2/3
  Switch1/1 -> Switch2/1
  [body_z] -> Cross Product2/2

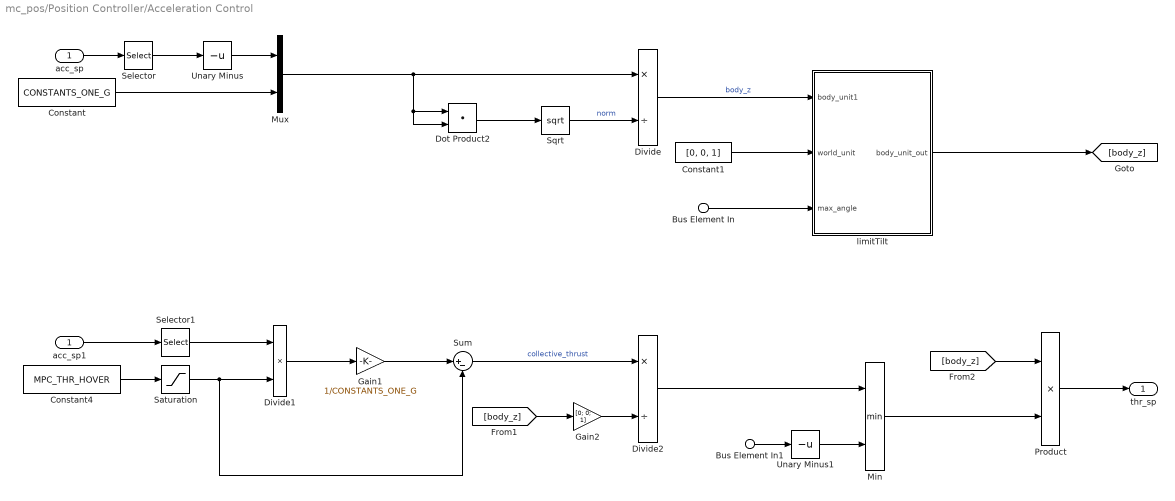
== system mc_pos/Position Controller/Acceleration Control ==
  acc_sp : Inport
  Bus Element In : Inport  Port=2  PortName=limit  Element=lim_tilt
  Bus Element In1 : Inport  Port=2  PortName=limit  Element=lim_thr_min
  Constant : Constant  Value=CONSTANTS_ONE_G  OutDataTypeStr=single
  Constant1 : Constant  Value=[0, 0, 1]  OutDataTypeStr=single
  Constant4 : Constant  Value=MPC_THR_HOVER  OutDataTypeStr=single
  Divide : Product  Inputs=*/
  Divide1 : Product  Inputs=**
  Divide2 : Product  Inputs=*/
  Dot Product2 : DotProduct  InputSameDT=on  OutDataTypeStr=Inherit: Inherit via internal rule
  Gain1 : Gain  Gain=1/CONSTANTS_ONE_G
      settings: AttributesFormatString=%<Gain>
  Gain2 : Gain  Gain=[0; 0; 1]
      settings: AttributesFormatString=%<Gain>
  Min : MinMax  Inputs=2
  Mux : Mux  Inputs=2
  Product : Product
  Saturation : Saturate  UpperLimit=0.9  LowerLimit=0.1  OutDataTypeStr=single
      settings: AttributesFormatString=[%<LowerLimit>, %<UpperLimit>]
  Selector : Selector  InputPortWidth=3  IndexOptions=Index vector (dialog)  Indices=[1 2]  OutputSizes=1
  Selector1 : Selector  InputPortWidth=3  IndexOptions=Index vector (dialog)  Indices=3  OutputSizes=1
  Sqrt : Sqrt  SaturateOnIntegerOverflow=on
  Sum : Sum  Inputs=|+-
  Unary Minus : UnaryMinus
  Unary Minus1 : UnaryMinus
  acc_sp1 : InportShadow
  limitTilt : Subsystem
  thr_sp : Outport
  wires:
  acc_sp/1 -> Selector/1
  Selector/1 -> Unary Minus/1
  Unary Minus/1 -> Mux/1
  Constant/1 -> Mux/2
  Mux/1 -> Dot Product2/2, Dot Product2/1, Divide/1
  Sqrt/1 -> Divide/2  "norm"
  Divide/1 -> limitTilt/1(body_unit1)  "body_z"
  Dot Product2/1 -> Sqrt/1
  Bus Element In/1 -> limitTilt/3(max_angle)
  Constant1/1 -> limitTilt/2(world_unit)
  limitTilt/1(body_unit_out) -> [body_z]
  acc_sp1/1 -> Selector1/1
  Divide1/1 -> Gain1/1
  Sum/1 -> Divide2/1  "collective_thrust"
  [body_z] -> Gain2/1
  Gain2/1 -> Divide2/2
  Divide2/1 -> Min/1
  Unary Minus1/1 -> Min/2
  Bus Element In1/1 -> Unary Minus1/1
  Min/1 -> Product/2
  [body_z] -> Product/1
  Product/1 -> thr_sp/1
  Constant4/1 -> Saturation/1
  Saturation/1 -> Sum/2, Divide1/2
  Selector1/1 -> Divide1/1
  Gain1/1 -> Sum/1

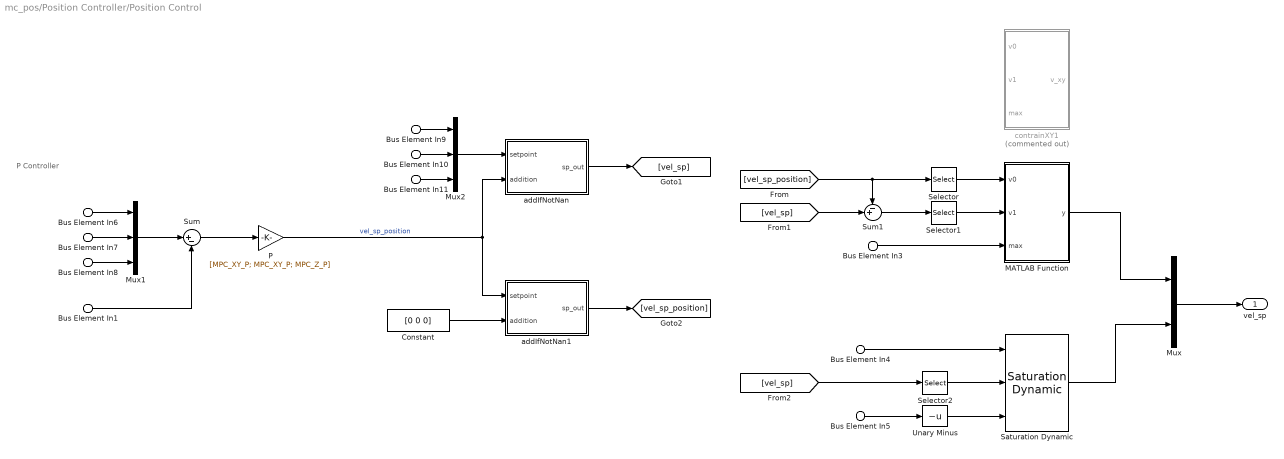
== system mc_pos/Position Controller/Position Control ==
  note: P Controller
  Bus Element In6 : Inport  PortName=setpoint  Element=x
  Bus Element In7 : Inport  PortName=setpoint  Element=y
  Bus Element In8 : Inport  PortName=setpoint  Element=z
  Bus Element In9 : Inport  PortName=setpoint  Element=vx
  Bus Element In10 : Inport  PortName=setpoint  Element=vy
  Bus Element In11 : Inport  PortName=setpoint  Element=vz
  Bus Element In1 : Inport  Port=2  PortName=state  Element=pos
  Bus Element In3 : Inport  Port=3  PortName=limit  Element=lim_vel_horizontal
  Bus Element In4 : Inport  Port=3  PortName=limit  Element=lim_vel_down
  Bus Element In5 : Inport  Port=3  PortName=limit  Element=lim_vel_up
  Constant : Constant  Value=[0 0 0]  OutDataTypeStr=single
  MATLAB Function : MATLAB Function  TreatAsAtomicUnit=on
  Mux : Mux  Inputs=2
  Mux1 : Mux  Inputs=3
  Mux2 : Mux  Inputs=3
  P : Gain  Gain=[MPC_XY_P; MPC_XY_P; MPC_Z_P]
      settings: AttributesFormatString=%<Gain>
  Saturation Dynamic : simulink/Discontinuities/Saturation Dynamic  OutMin=[]  OutMax=[]  OutDataTypeStr=Inherit: Same as second input  OutDataType=fixdt(1, 16)  OutScaling=2^-10  DoSatur=off
  Selector : Selector  InputPortWidth=3  IndexOptions=Index vector (dialog)  Indices=[1 2]  OutputSizes=1
  Selector1 : Selector  InputPortWidth=3  IndexOptions=Index vector (dialog)  Indices=[1 2]  OutputSizes=1
  Selector2 : Selector  InputPortWidth=3  IndexOptions=Index vector (dialog)  Indices=3  OutputSizes=1
  Sum : Sum  Inputs=|+-
  Sum1 : Sum  Inputs=-+|
  Unary Minus : UnaryMinus
  addIfNotNan : Subsystem
  addIfNotNan1 : Subsystem
  contrainXY1 : Subsystem  Commented=on
  vel_sp : Outport
  wires:
  Mux1/1 -> Sum/1
  Bus Element In1/1 -> Sum/2
  Sum/1 -> P/1
  P/1 -> addIfNotNan1/1(setpoint), addIfNotNan/2(addition)  "vel_sp_position"
  Mux2/1 -> addIfNotNan/1(setpoint)
  addIfNotNan/1(sp_out) -> [vel_sp]
  Constant/1 -> addIfNotNan1/2(addition)
  addIfNotNan1/1(sp_out) -> [vel_sp_position]
  [vel_sp_position] -> Sum1/1, Selector/1
  Selector/1 -> MATLAB Function/1(v0)
  Bus Element In3/1 -> MATLAB Function/3(max)
  [vel_sp] -> Sum1/2
  Sum1/1 -> Selector1/1
  Selector1/1 -> MATLAB Function/2(v1)
  [vel_sp] -> Selector2/1
  Selector2/1 -> Saturation Dynamic/2
  Bus Element In4/1 -> Saturation Dynamic/1
  Unary Minus/1 -> Saturation Dynamic/3
  Bus Element In5/1 -> Unary Minus/1
  Saturation Dynamic/1 -> Mux/2
  MATLAB Function/1(y) -> Mux/1
  Mux/1 -> vel_sp/1
  Bus Element In6/1 -> Mux1/1
  Bus Element In7/1 -> Mux1/2
  Bus Element In8/1 -> Mux1/3
  Bus Element In9/1 -> Mux2/1
  Bus Element In10/1 -> Mux2/2
  Bus Element In11/1 -> Mux2/3

== system mc_pos/Position Controller/Velocity Control ==
  Bus Element In : Inport  PortName=state  Element=vel
  Bus Element In1 : Inport  PortName=state  Element=vel_dot
  vel_sp : Inport  Port=2
  acc_sp : Inport  Port=3
  Bus Element In2 : Inport  Port=4  PortName=limit
  reset : Inport  Port=5
  last_thr_sp : Inport  Port=6
  D : Gain  Gain=[MPC_XY_VEL_D_ACC; MPC_XY_VEL_D_ACC; MPC_Z_VEL_D_ACC]
      settings: AttributesFormatString=%<Gain>
  Delay One Step : Delay  DelayLength=1
  I : Subsystem
  P : Gain  Gain=[MPC_XY_VEL_P_ACC; MPC_XY_VEL_P_ACC; MPC_Z_VEL_P_ACC]
      settings: AttributesFormatString=%<Gain>
  Sum : Sum  Inputs=|+-
  Sum1 : Sum  Inputs=++-
  addIfNotNan : Subsystem
  acc_sp_out : Outport
  wires:
  Sum/1 -> P/1, I/1(vel_error)
  P/1 -> Sum1/1
  D/1 -> Sum1/3
  Bus Element In1/1 -> D/1
  Bus Element In/1 -> Sum/2
  I/1(vel_init) -> Sum1/2
  vel_sp/1 -> Sum/1
  Sum1/1 -> addIfNotNan/2(addition)  "acc_sp_velocity"
  Bus Element In2/1 -> I/4(limit)
  acc_sp/1 -> addIfNotNan/1(setpoint)
  addIfNotNan/1(sp_out) -> Delay One Step/1, acc_sp_out/1
  [acc_sp] -> I/2(acc_sp)
  last_thr_sp/1 -> I/3(last_thr_sp)
  reset/1 -> I/5(reset)
  Delay One Step/1 -> [acc_sp]

== system mc_pos/Position Controller/limitation ==
  thr_sp : Inport
  lim_thr_max : Inport  Port=2
  Constant : Constant  Value=0  OutDataTypeStr=single
  Divide : Product  Inputs=*/*
  Dot Product1 : DotProduct  InputSameDT=on  OutDataTypeStr=Inherit: Inherit via internal rule
  Math Function : Math  Operator=square  SaturateOnIntegerOverflow=on
  Math Function1 : Math  Operator=square  SaturateOnIntegerOverflow=on
  Max : MinMax  Function=max  Inputs=2
  Mux : Mux  Inputs=2
  Saturation : Saturate  UpperLimit=inf  LowerLimit=0
      settings: AttributesFormatString=[%<LowerLimit>, %<UpperLimit>]
  Saturation Dynamic : simulink/Discontinuities/Saturation Dynamic  OutMin=[]  OutMax=[]  OutDataTypeStr=Inherit: Same as second input  OutDataType=fixdt(1, 16)  OutScaling=2^-10  DoSatur=off
  Selector : Selector  InputPortWidth=3  IndexOptions=Index vector (dialog)  Indices=[1 2]  OutputSizes=1
  Selector1 : Selector  InputPortWidth=3  IndexOptions=Index vector (dialog)  Indices=3  OutputSizes=1
  Sqrt : Sqrt  SaturateOnIntegerOverflow=on
  Sqrt1 : Sqrt  SaturateOnIntegerOverflow=on
  Sum : Sum  Inputs=|+-
  Unary Minus : UnaryMinus
  thr_sp1 : InportShadow
  thr_sp_out : Outport
  wires:
  thr_sp/1 -> Selector1/1
  lim_thr_max/1 -> Math Function/1, Unary Minus/1
  Selector1/1 -> Max/1
  Unary Minus/1 -> Max/2
  Max/1 -> [thr_sp_z]
  Math Function/1 -> Sum/1  "thrust_max_squared"
  [thr_sp_z] -> Math Function1/1
  Math Function1/1 -> Sum/2  "thrust_z_squared"
  Sum/1 -> Saturation/1  "thrust_max_xy_squared"
  Saturation/1 -> Sqrt/1
  Sqrt/1 -> [thrust_max_xy]
  thr_sp1/1 -> Selector/1
  Selector/1 -> Dot Product1/2, Dot Product1/1, Divide/1
  Dot Product1/1 -> Sqrt1/1
  Sqrt1/1 -> Saturation Dynamic/2, Divide/2  "thrust_sp_xy_norm"
  Saturation Dynamic/1 -> Divide/3
  [thrust_max_xy] -> Saturation Dynamic/1
  Constant/1 -> Saturation Dynamic/3
  Divide/1 -> [thr_sp_xy]
  Mux/1 -> thr_sp_out/1
  [thr_sp_xy] -> Mux/1
  [thr_sp_z] -> Mux/2

== system mc_pos/Position Controller/updateSuccessful ==
  Bus Element In : Inport  PortName=setpoint  Element=pos_sp
  Bus Element In1 : Inport  PortName=setpoint  Element=vel_sp
  Bus Element In2 : Inport  PortName=setpoint  Element=acc_sp
  AND : Logic  Inputs=3  AllPortsSameDT=off  OutDataTypeStr=boolean
  Relational Operator : RelationalOperator  Operator===  OutDataTypeStr=boolean  RndMeth=Simplest
  Relational Operator1 : RelationalOperator  Operator===  OutDataTypeStr=boolean  RndMeth=Simplest
  Relational Operator2 : RelationalOperator  Operator===  OutDataTypeStr=boolean  RndMeth=Simplest
  Selector : Selector  InputPortWidth=3  IndexOptions=Index vector (dialog)  Indices=1  OutputSizes=1
  Selector1 : Selector  InputPortWidth=3  IndexOptions=Index vector (dialog)  Indices=2  OutputSizes=1
  Selector2 : Selector  InputPortWidth=3  IndexOptions=Index vector (dialog)  Indices=1  OutputSizes=1
  Selector3 : Selector  InputPortWidth=3  IndexOptions=Index vector (dialog)  Indices=2  OutputSizes=1
  Selector4 : Selector  InputPortWidth=3  IndexOptions=Index vector (dialog)  Indices=1  OutputSizes=1
  Selector5 : Selector  InputPortWidth=3  IndexOptions=Index vector (dialog)  Indices=2  OutputSizes=1
  wires:
  Relational Operator1/1 -> AND/2
  Selector1/1 -> Relational Operator/2
  Selector4/1 -> Relational Operator2/1
  Relational Operator/1 -> AND/1
  Relational Operator2/1 -> AND/3
  Selector5/1 -> Relational Operator2/2
  Selector3/1 -> Relational Operator1/2
  AND/1 -> [valid]
  Selector2/1 -> Relational Operator1/1
  Selector/1 -> Relational Operator/1
  Bus Element In/1 -> Selector1/1, Selector/1
  Bus Element In1/1 -> Selector3/1, Selector2/1
  Bus Element In2/1 -> Selector5/1, Selector4/1

== system mc_pos/Update States/lowpass filter ==
  note: lowpass filter
  input : Inport
  Constant : Constant  OutDataTypeStr=single
  Constant3 : Constant  Value=MPC_VELD_LP  OutDataTypeStr=single
  Constant4 : Constant  OutDataTypeStr=single
  Constant5 : Constant  OutDataTypeStr=single
  Delay One Step : Delay  DelayLength=1
  Divide : Product  Inputs=*/
  Gain : Gain  Gain=2*pi
  Product : Product
  Product1 : Product
  Product2 : Product
  Sum : Sum  Inputs=++|
  Sum1 : Sum  Inputs=+-
  Sum2 : Sum  Inputs=++|
  Weighted Sample Time : SampleTimeMath  TsampMathOp=Ts Only
  state : Outport
  wires:
  input/1 -> Product/2
  Product/1 -> Sum/2
  Sum/1 -> Delay One Step/1, state/1
  Product1/1 -> Sum/1
  Delay One Step/1 -> Product1/2
  Divide/1 -> Sum1/2, Product/1  "a"
  Sum1/1 -> Product1/1
  Constant/1 -> Sum1/1
  Product2/1 -> Sum2/1, Divide/1  "b"
  Sum2/1 -> Divide/2
  Constant4/1 -> Sum2/2
  Constant3/1 -> Gain/1
  Constant5/1 -> Weighted Sample Time/1
  Gain/1 -> Product2/1
  Weighted Sample Time/1 -> Product2/2

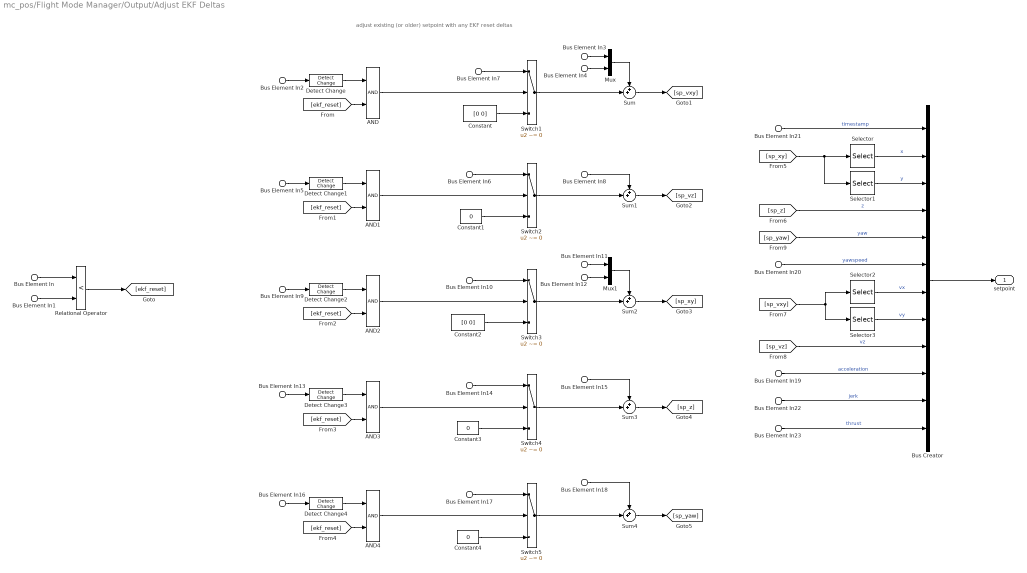
== system mc_pos/Flight Mode Manager/Output/Adjust EKF Deltas ==
  note: adjust existing (or older) setpoint with any EKF reset deltas
  Bus Element In1 : Inport  PortName=local_pos  Element=timestamp
  Bus Element In2 : Inport  PortName=local_pos  Element=vxy_reset_counter
  Bus Element In7 : Inport  PortName=local_pos  Element=delta_vxy
  Bus Element In5 : Inport  PortName=local_pos  Element=vz_reset_counter
  Bus Element In6 : Inport  PortName=local_pos  Element=delta_vz
  Bus Element In9 : Inport  PortName=local_pos  Element=xy_reset_counter
  Bus Element In10 : Inport  PortName=local_pos  Element=delta_xy
  Bus Element In13 : Inport  PortName=local_pos  Element=z_reset_counter
  Bus Element In14 : Inport  PortName=local_pos  Element=delta_z
  Bus Element In16 : Inport  PortName=local_pos  Element=heading_reset_counter
  Bus Element In17 : Inport  PortName=local_pos  Element=delta_heading
  Bus Element In : Inport  Port=2  PortName=traj_sp  Element=timestamp
  Bus Element In21 : Inport  Port=2  PortName=traj_sp  Element=timestamp
  Bus Element In3 : Inport  Port=2  PortName=traj_sp  Element=vx
  Bus Element In4 : Inport  Port=2  PortName=traj_sp  Element=vy
  Bus Element In8 : Inport  Port=2  PortName=traj_sp  Element=vz
  Bus Element In11 : Inport  Port=2  PortName=traj_sp  Element=x
  Bus Element In12 : Inport  Port=2  PortName=traj_sp  Element=y
  Bus Element In15 : Inport  Port=2  PortName=traj_sp  Element=z
  Bus Element In18 : Inport  Port=2  PortName=traj_sp  Element=yaw
  Bus Element In19 : Inport  Port=2  PortName=traj_sp  Element=acceleration
  Bus Element In20 : Inport  Port=2  PortName=traj_sp  Element=yawspeed
  Bus Element In22 : Inport  Port=2  PortName=traj_sp  Element=jerk
  Bus Element In23 : Inport  Port=2  PortName=traj_sp  Element=thrust
  AND{,1..4} (5 alike) : Logic  AllPortsSameDT=off  OutDataTypeStr=boolean
  Bus Creator : BusCreator  Inputs=12
  Constant : Constant  Value=[0 0]  OutDataTypeStr=single
  Constant1 : Constant  Value=0  OutDataTypeStr=single
  Constant2 : Constant  Value=[0 0]  OutDataTypeStr=single
  Constant3 : Constant  Value=0  OutDataTypeStr=single
  Constant4 : Constant  Value=0  OutDataTypeStr=single
  Detect Change{,1..4} (5 alike) : simulink/Logic and Bit Operations/Detect Change  vinit=0  OutDataTypeStr=boolean
  Mux : Mux  Inputs=2
  Mux1 : Mux  Inputs=2
  Relational Operator : RelationalOperator  Operator=<  OutDataTypeStr=boolean  RndMeth=Simplest
  Selector : Selector  InputPortWidth=2  IndexOptions=Index vector (dialog)  Indices=1  OutputSizes=1
  Selector1 : Selector  InputPortWidth=2  IndexOptions=Index vector (dialog)  Indices=2  OutputSizes=1
  Selector2 : Selector  InputPortWidth=2  IndexOptions=Index vector (dialog)  Indices=1  OutputSizes=1
  Selector3 : Selector  InputPortWidth=2  IndexOptions=Index vector (dialog)  Indices=2  OutputSizes=1
  Sum{,1..4} (5 alike) : Sum  Inputs=++|
  Switch{1..5} (5 alike) : Switch  Criteria=u2 ~= 0
  setpoint : Outport
  wires:
  Bus Element In/1 -> Relational Operator/1
  Bus Element In1/1 -> Relational Operator/2
  Relational Operator/1 -> [ekf_reset]
  Bus Element In2/1 -> Detect Change/1
  Detect Change/1 -> AND/1
  [ekf_reset] -> AND/2
  AND/1 -> Switch1/2
  Constant/1 -> Switch1/3
  Bus Element In3/1 -> Mux/1
  Bus Element In4/1 -> Mux/2
  Bus Element In7/1 -> Switch1/1
  Switch1/1 -> Sum/2
  Mux/1 -> Sum/1
  Sum/1 -> [sp_vxy]
  Bus Element In5/1 -> Detect Change1/1
  Detect Change1/1 -> AND1/1
  [ekf_reset] -> AND1/2
  AND1/1 -> Switch2/2
  Bus Element In6/1 -> Switch2/1
  Constant1/1 -> Switch2/3
  Switch2/1 -> Sum1/2
  Bus Element In8/1 -> Sum1/1
  Sum1/1 -> [sp_vz]
  Bus Element In9/1 -> Detect Change2/1
  Detect Change2/1 -> AND2/1
  [ekf_reset] -> AND2/2
  AND2/1 -> Switch3/2
  Bus Element In10/1 -> Switch3/1
  Constant2/1 -> Switch3/3
  Switch3/1 -> Sum2/2
  Mux1/1 -> Sum2/1
  Bus Element In11/1 -> Mux1/1
  Bus Element In12/1 -> Mux1/2
  Sum2/1 -> [sp_xy]
  Bus Element In13/1 -> Detect Change3/1
  [ekf_reset] -> AND3/2
  Detect Change3/1 -> AND3/1
  AND3/1 -> Switch4/2
  Bus Element In14/1 -> Switch4/1
  Constant3/1 -> Switch4/3
  Switch4/1 -> Sum3/2
  Bus Element In15/1 -> Sum3/1
  Sum3/1 -> [sp_z]
  Bus Element In16/1 -> Detect Change4/1
  Detect Change4/1 -> AND4/1
  [ekf_reset] -> AND4/2
  AND4/1 -> Switch5/2
  Constant4/1 -> Switch5/3
  Bus Element In17/1 -> Switch5/1
  Switch5/1 -> Sum4/2
  Bus Element In18/1 -> Sum4/1
  Sum4/1 -> [sp_yaw]
  Bus Creator/1 -> setpoint/1
  [sp_xy] -> Selector1/1, Selector/1
  Selector/1 -> Bus Creator/2  "x"
  Selector1/1 -> Bus Creator/3  "y"
  [sp_z] -> Bus Creator/4  "z"
  [sp_vxy] -> Selector2/1, Selector3/1
  Selector2/1 -> Bus Creator/7  "vx"
  Selector3/1 -> Bus Creator/8  "vy"
  [sp_vz] -> Bus Creator/9  "vz"
  Bus Element In19/1 -> Bus Creator/10  "acceleration"
  [sp_yaw] -> Bus Creator/5  "yaw"
  Bus Element In20/1 -> Bus Creator/6  "yawspeed"
  Bus Element In21/1 -> Bus Creator/1  "timestamp"
  Bus Element In22/1 -> Bus Creator/11  "jerk"
  Bus Element In23/1 -> Bus Creator/12  "thrust"

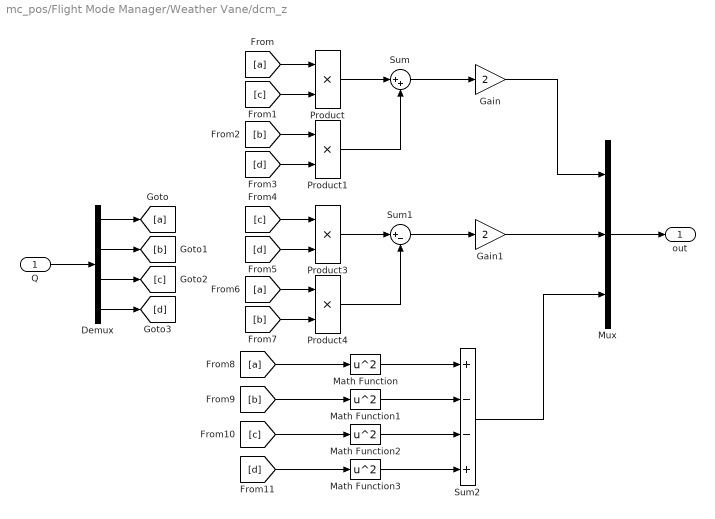
== system mc_pos/Flight Mode Manager/Weather Vane/dcm_z ==
  Q : Inport
  Demux : Demux
  Gain : Gain  Gain=2  OutDataTypeStr=single
  Gain1 : Gain  Gain=2  OutDataTypeStr=single
  Math Function{,1..3} (4 alike) : Math  Operator=square  SaturateOnIntegerOverflow=on
  Mux : Mux  Inputs=3
  Product{,1,3..4} (4 alike) : Product
  Sum : Sum  Inputs=|++
  Sum1 : Sum  Inputs=|+-
  Sum2 : Sum  Inputs=+--+
  out : Outport
  wires:
  Q/1 -> Demux/1
  Demux/1 -> [a]
  Demux/2 -> [b]
  Demux/3 -> [c]
  Demux/4 -> [d]
  [a] -> Product/1
  [c] -> Product/2
  Product/1 -> Sum/1
  [b] -> Product1/1
  [d] -> Product1/2
  Product1/1 -> Sum/2
  Sum/1 -> Gain/1
  Mux/1 -> out/1
  [c] -> Product3/1
  [d] -> Product3/2
  Product3/1 -> Sum1/1
  [a] -> Product4/1
  [b] -> Product4/2
  Product4/1 -> Sum1/2
  Sum2/1 -> Mux/3
  [a] -> Math Function/1
  [b] -> Math Function1/1
  [c] -> Math Function2/1
  [d] -> Math Function3/1
  Math Function/1 -> Sum2/1
  Math Function1/1 -> Sum2/2
  Math Function2/1 -> Sum2/3
  Math Function3/1 -> Sum2/4
  Gain/1 -> Mux/1
  Gain1/1 -> Mux/2
  Sum1/1 -> Gain1/1

== system mc_pos/Position Controller/Acceleration Control/limitTilt ==
  body_unit1 : Inport
  world_unit : Inport  Port=2
  max_angle : Inport  Port=3
  Acos : Trigonometry  Operator=acos
  Constant : Constant  OutDataTypeStr=single
  Cos : Trigonometry  Operator=cos
  Cos1 : Trigonometry
  Divide : Product  Inputs=*/
  Dot Product : DotProduct  InputSameDT=on  OutDataTypeStr=Inherit: Inherit via internal rule
  Dot Product1 : DotProduct  InputSameDT=on  OutDataTypeStr=Inherit: Inherit via internal rule
  Dot Product3 : DotProduct  InputSameDT=on  OutDataTypeStr=Inherit: Inherit via internal rule
  Min : MinMax  Inputs=2
  Mux : Mux  Inputs=2
  Product1 : Product
  Product2 : Product
  Product3 : Product
  Selector1 : Selector  InputPortWidth=3  IndexOptions=Index vector (dialog)  Indices=[2 3]  OutputSizes=1
  Sqrt : Sqrt  SaturateOnIntegerOverflow=on
  Sum : Sum  Inputs=|+-
  Sum1 : Sum  Inputs=|++
  Switch : Switch  Threshold=eps
      settings: AttributesFormatString=|
      | %<Criteria>
      | %<Threshold>
  body_unit : InportShadow
  world_unit1 : InportShadow  Port=2
  body_unit_out : Outport
  wires:
  world_unit/1 -> Dot Product/1, Product3/1
  Dot Product/1 -> Product3/2, Acos/1  "dot_product_unit"
  Acos/1 -> Min/1
  max_angle/1 -> Min/2
  Min/1 -> [angle]
  Sum/1 -> Selector1/1, Dot Product1/2, Dot Product1/1, Switch/1  "rejection"
  Dot Product1/1 -> Switch/2
  Constant/1 -> Mux/1
  Selector1/1 -> Mux/2
  Mux/1 -> Switch/3
  [angle] -> Cos/1
  Cos/1 -> Product1/1
  world_unit1/1 -> Product1/2
  Product1/1 -> Sum1/1
  [angle] -> Cos1/1
  Cos1/1 -> Product2/1
  Product2/1 -> Sum1/2
  Switch/1 -> Divide/1, Dot Product3/2, Dot Product3/1  "rejection"
  Dot Product3/1 -> Sqrt/1
  Sqrt/1 -> Divide/2  "norm"
  Divide/1 -> Product2/2
  Sum1/1 -> body_unit_out/1
  body_unit/1 -> Sum/1
  Product3/1 -> Sum/2
  body_unit1/1 -> Dot Product/2
